simulink model "FiboSimulink_StateflowChart"  (R2025b)
settings: Solver=FixedStepDiscrete  StartTime=0.0  StopTime=0.9  FixedStep=1  RelTol=1e-3
undefined symbols (not defined in the file or in its folder): n
settings Model: Creator=marcu  LastModifiedBy=lucas
settings DataIOCC: SaveOutput=off  DSMLogging=off  SaveTime=off  ReturnWorkspaceOutputs=off  SignalLoggingName=FiboSimulink_StateflowChart_nthFiboNumber

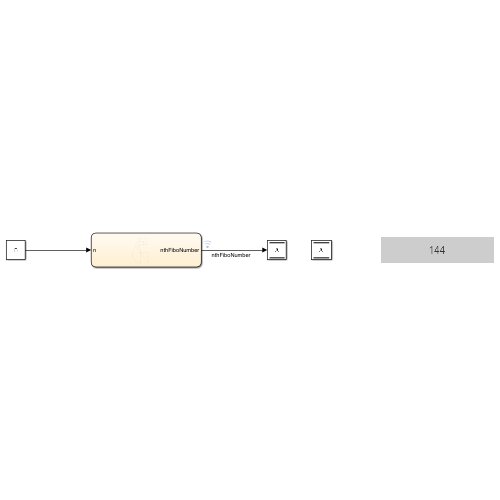
[thumbnail: Simulink's stored preview of the top-level diagram]
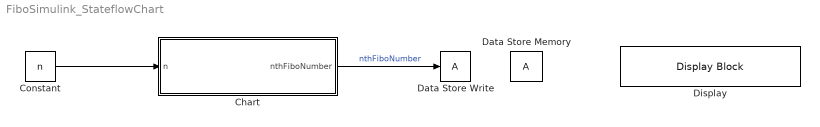
== system FiboSimulink_StateflowChart ==
  Chart : Stateflow chart  TreatAsAtomicUnit=on
  Constant : Constant  Value=n
  Data Store Memory : DataStoreMemory  WriteAfterWriteMsg=warning  ShowAdditionalParam=off
  Data Store Write : DataStoreWrite  IndexOptions=Index vector (dialog)  Indices=1  OutputSizes=1
  Display : DisplayBlock  LabelPosition=Hide  Transparency=1  GridColor=[0.502, 0.502, 0.502]
  wires:
  Constant/1 -> Chart/1(n)
  Chart/1(nthFiboNumber) -> Data Store Write/1  "nthFiboNumber"

== stateflow chart FiboSimulink_StateflowChart/Chart ==
  (default) -> (junction 13) : % Start condition
  (junction 13) -> (junction 14) [order 1] : [n == 0]
  (junction 13) -> (junction 15) [order 2]
  (junction 14) -> (junction 19) : {nthFiboNumber = 0;}
  (junction 15) -> (junction 16) [order 1] : [n == 1]
  (junction 15) -> (junction 28) [order 2]
  (junction 16) -> (junction 18) : {nthFiboNumber = 1;}
  (junction 18) -> (junction 17)
  (junction 19) -> (junction 18)
  (junction 33) -> (junction 17)
  (junction 17) -> (junction 20)
  (junction 28) -> (junction 30) : {i=0; F1=0; F2=1;}
  (junction 30) -> (junction 29) [order 1] : [i<n-1]
  (junction 29) -> (junction 31) : {nthFiboNumber = F1 + F2; F1 = F2; F2 = nthFiboNumber}
  (junction 32) -> (junction 30)
  (junction 30) -> (junction 33) [order 2]
  (junction 31) -> (junction 32) : {i=i+1;}
  data: n input; nthFiboNumber output; i local; F1 local; F2 local
